simulink model "DrivetrainEv_3motor_PTBS"  (R2020a)
settings: configuration reference "Config_VarStep_Long" (kept outside this file)
undefined symbols (not defined in the file): b, b_CG, br, g, k, Mass, Ndiff_rear, NF, NR, T
libraries: autolibshared x11, autolibsharedcoupling x5, autolibcoupling x2, autolibutils x2, autolibshareddiff x1
(part 1 of 6)
settings Model: DataDictionary=System_Data_Dictionary.sldd  ModifiedByFormat=The MathWorks, Inc.  PauseTimes=10  Creator=The MathWorks, Inc.  LastModifiedBy=The MathWorks, Inc.
settings ConfigSetRef: SourceName=Config_VarStep_Long

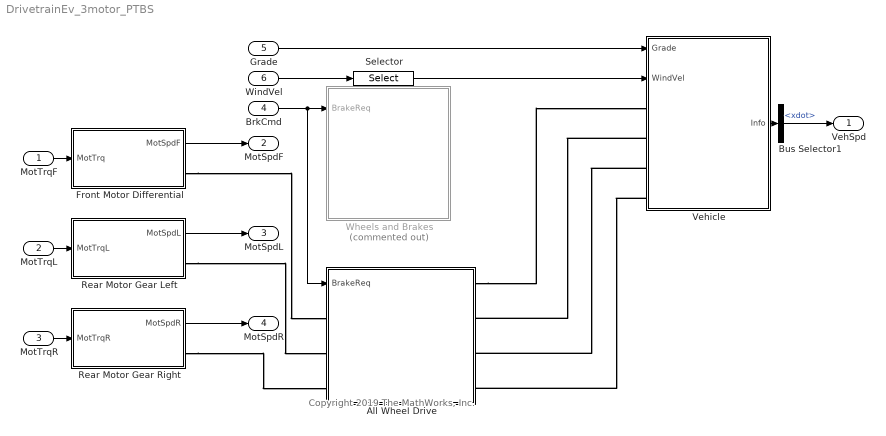
== system DrivetrainEv_3motor_PTBS ==
  note: Copyright 2019 The MathWorks, Inc.
  MotTrqF : Inport
  MotTrqL : Inport  Port=2
  MotTrqR : Inport  Port=3
  BrkCmd : Inport  Port=4
  Grade : Inport  Port=5
  WindVel : Inport  Port=6
  All Wheel Drive : Subsystem  VariantControl=2
  Bus Selector1 : BusSelector  OutputSignals=BdyFrm.Cg.Vel.xdot
  Front Motor Differential : Subsystem  VariantControl=0
  Rear Motor Gear Left : Subsystem  VariantControl=0
  Rear Motor Gear Right : Subsystem  VariantControl=0
  Selector : Selector  InputPortWidth=3  IndexOptions=Index vector (dialog)  Indices=[1]  OutputSizes=1
  Vehicle : Subsystem
  Wheels and Brakes : Subsystem  Commented=on  Variant=on  VariantControlMode=Label  LabelModeActiveChoice=2
  VehSpd : Outport  VectorParamsAs1DForOutWhenUnconnected=off
  MotSpdF : Outport  Port=2  VectorParamsAs1DForOutWhenUnconnected=off  BusOutputAsStruct=on
  MotSpdL : Outport  Port=3  VectorParamsAs1DForOutWhenUnconnected=off  BusOutputAsStruct=on
  MotSpdR : Outport  Port=4  VectorParamsAs1DForOutWhenUnconnected=off  BusOutputAsStruct=on
  wires:
  Rear Motor Gear Left/1(MotSpdL) -> MotSpdL/1
  Rear Motor Gear Right/1(MotSpdR) -> MotSpdR/1
  MotTrqL/1 -> Rear Motor Gear Left/1(MotTrqL)
  MotTrqR/1 -> Rear Motor Gear Right/1(MotTrqR)
  WindVel/1 -> Selector/1
  BrkCmd/1 -> All Wheel Drive/1(BrakeReq), Wheels and Brakes/1(BrakeReq)
  Grade/1 -> Vehicle/1(Grade)
  Bus Selector1/1 -> VehSpd/1  "<xdot>"
  Vehicle/1(Info) -> Bus Selector1/1
  Selector/1 -> Vehicle/2(WindVel)
  Front Motor Differential/1(MotSpdF) -> MotSpdF/1
  MotTrqF/1 -> Front Motor Differential/1(MotTrq)
  connections:
  Front Motor Differential/RConn1 -- All Wheel Drive/LConn1
  Rear Motor Gear Left/RConn1 -- All Wheel Drive/LConn2
  Rear Motor Gear Right/RConn1 -- All Wheel Drive/LConn3
  All Wheel Drive/RConn1 -- Vehicle/LConn1
  Vehicle/LConn2 -- All Wheel Drive/RConn2
  Vehicle/LConn3 -- All Wheel Drive/RConn3
  Vehicle/LConn4 -- All Wheel Drive/RConn4
